simulink model "simulation"  (R2020a)
settings: Solver=VariableStepAuto  StartTime=0.0  StopTime=1200  RelTol=1e-3
values from neighbouring files (symbols this model uses):
  CHR1_Kp = 0.6/k/a    (= 0.258906601048)    [code.m]
  CHR1_Td = 0.5*Td    (= 7.8)    [code.m]
  CHR1_Ti = Td    (= 15.6)    [code.m]
  CHR2_Kp = 0.95/k/a    (= 0.40993545166)    [code.m]
  CHR2_Td = 0.42*Td    (= 6.552)    [code.m]
  CHR2_Ti = 2.38*Td    (= 37.128)    [code.m]
  k = 7.19    [code.m]
  T = 48.4    [code.m]
  Td = 15.6    [code.m]
  ZN_Kp = 1.2/k/a    (= 0.517813202097)    [code.m]
  ZN_Td = 0.5*Td    (= 7.8)    [code.m]
  ZN_Ti = 2*Td    (= 31.2)    [code.m]
undefined symbols (not defined in the file or in its folder): sigbuilder_block
settings Model: Creator=AMIRHOSEIN  LastModifiedBy=AMIRHOSEIN

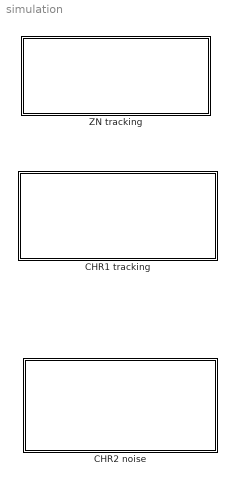
== system simulation ==
  CHR1 tracking : Subsystem
  CHR2 noise : Subsystem
  ZN tracking : Subsystem

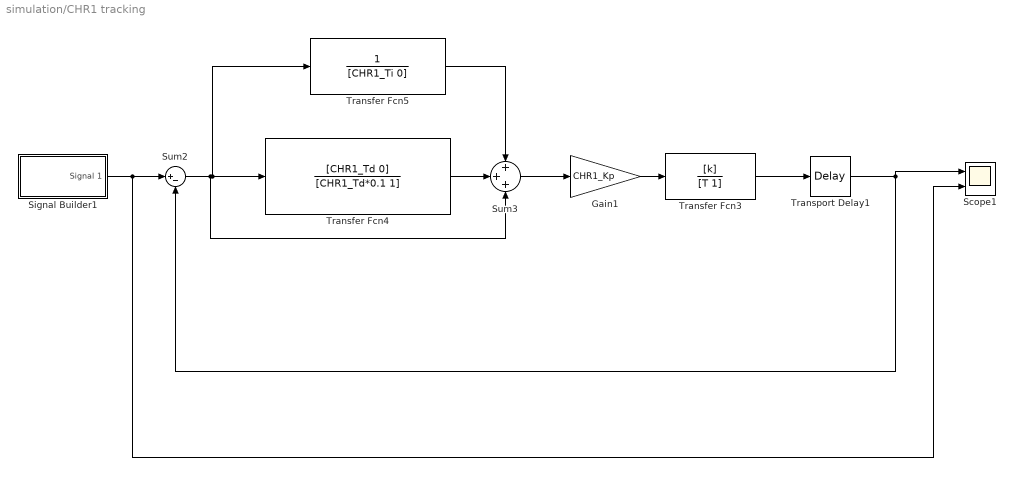
== system simulation/CHR1 tracking ==
  Gain1 : Gain  Gain=CHR1_Kp
  Scope1 : Scope  NumInputPorts=2
  Signal Builder1 : Subsystem  Tag=STV Subsys  LoadFcn=sigbuilder_block('load');  StartFcn=sigbuilder_block('start');  StopFcn=sigbuilder_block('stop');  ClipboardFcn=sigbuilder_block('clipboard');  mask(Sigbuilder block){tuvar=[0:10]}
      mask help: Simulink:masks:SigbuilderBlock_MD
      mask init:
      | if ~strcmp(get_param(bdroot(gcbh),'SimulationStatus'),'stopped') tuvar = sigbuilder_block('maskInit'); end
      settings: CopyFcn=sigbuilder_block('copy');  DeleteFcn=sigbuilder_block('delete');  ModelCloseFcn=sigbuilder_block('modelClose');  PreSaveFcn=sigbuilder_block('preSave');  PauseFcn=sigbuilder_block('pause');  ContinueFcn=sigbuilder_block('continue');  NameChangeFcn=sigbuilder_block('namechange');  OpenFcn=sigbuilder_block('open',[744.75 240 550.5 396 ]);  CloseFcn=sigbuilder_block('close');
      mask Display: plot(0, 0, 100, 100,[2, 2, 32, 32, 2], [68, 8, 8, 68, 68],[32, 2], [38, 38], [32, 19, 2],[53, 60, 44], [32, 17, 17, 2],[16, 16, 31, 31]);txt = getActiveGroup(gcbh);text(2, 100, txt,'verticalAlignment', 'top');
  Sum2 : Sum  Inputs=|+-
  Sum3 : Sum  Inputs=+++
  Transfer Fcn3 : TransferFcn  Numerator=[k]  Denominator=[T 1]
  Transfer Fcn4 : TransferFcn  Numerator=[CHR1_Td 0]  Denominator=[CHR1_Td*0.1 1]
  Transfer Fcn5 : TransferFcn  Denominator=[CHR1_Ti 0]
  Transport Delay1 : TransportDelay  DelayTime=Td
  wires:
  Transfer Fcn5/1 -> Sum3/1
  Transfer Fcn4/1 -> Sum3/2
  Transfer Fcn3/1 -> Transport Delay1/1
  Transport Delay1/1 -> Sum2/2, Scope1/1
  Sum2/1 -> Sum3/3, Transfer Fcn4/1, Transfer Fcn5/1
  Sum3/1 -> Gain1/1
  Gain1/1 -> Transfer Fcn3/1
  Signal Builder1/1(Signal 1) -> Scope1/2, Sum2/1

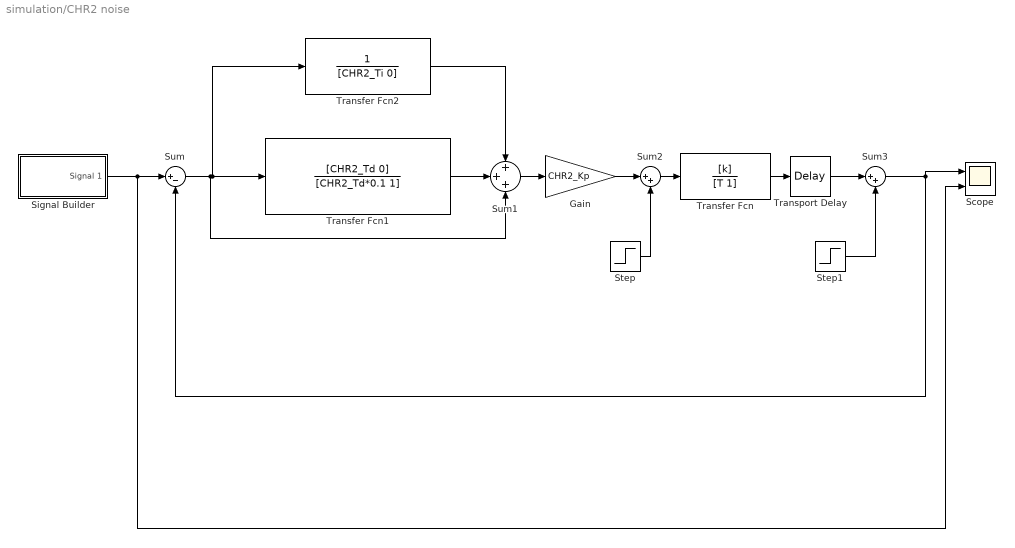
== system simulation/CHR2 noise ==
  Gain : Gain  Gain=CHR2_Kp
  Scope : Scope  NumInputPorts=2
  Signal Builder : Subsystem  Tag=STV Subsys  LoadFcn=sigbuilder_block('load');  StartFcn=sigbuilder_block('start');  StopFcn=sigbuilder_block('stop');  ClipboardFcn=sigbuilder_block('clipboard');  mask(Sigbuilder block){tuvar=[0:10]}
      mask help: Simulink:masks:SigbuilderBlock_MD
      mask init:
      | if ~strcmp(get_param(bdroot(gcbh),'SimulationStatus'),'stopped') tuvar = sigbuilder_block('maskInit'); end
      settings: CopyFcn=sigbuilder_block('copy');  DeleteFcn=sigbuilder_block('delete');  ModelCloseFcn=sigbuilder_block('modelClose');  PreSaveFcn=sigbuilder_block('preSave');  PauseFcn=sigbuilder_block('pause');  ContinueFcn=sigbuilder_block('continue');  NameChangeFcn=sigbuilder_block('namechange');  OpenFcn=sigbuilder_block('open',[538.5 220.5 550.5 396 ]);  CloseFcn=sigbuilder_block('close');
      mask Display: plot(0, 0, 100, 100,[2, 2, 32, 32, 2], [68, 8, 8, 68, 68],[32, 2], [38, 38], [32, 19, 2],[53, 60, 44], [32, 17, 17, 2],[16, 16, 31, 31]);txt = getActiveGroup(gcbh);text(2, 100, txt,'verticalAlignment', 'top');
  Step : Step  Time=600  After=10  SampleTime=0
  Step1 : Step  Time=1000  After=10  SampleTime=0
  Sum : Sum  Inputs=|+-
  Sum1 : Sum  Inputs=+++
  Sum2 : Sum  Inputs=|++
  Sum3 : Sum  Inputs=|++
  Transfer Fcn : TransferFcn  Numerator=[k]  Denominator=[T 1]
  Transfer Fcn1 : TransferFcn  Numerator=[CHR2_Td 0]  Denominator=[CHR2_Td*0.1 1]
  Transfer Fcn2 : TransferFcn  Denominator=[CHR2_Ti 0]
  Transport Delay : TransportDelay  DelayTime=Td
  wires:
  Signal Builder/1(Signal 1) -> Scope/2, Sum/1
  Step/1 -> Sum2/2
  Sum2/1 -> Transfer Fcn/1
  Sum3/1 -> Sum/2, Scope/1
  Transport Delay/1 -> Sum3/1
  Transfer Fcn/1 -> Transport Delay/1
  Gain/1 -> Sum2/1
  Step1/1 -> Sum3/2
  Sum/1 -> Sum1/3, Transfer Fcn1/1, Transfer Fcn2/1
  Transfer Fcn1/1 -> Sum1/2
  Transfer Fcn2/1 -> Sum1/1
  Sum1/1 -> Gain/1

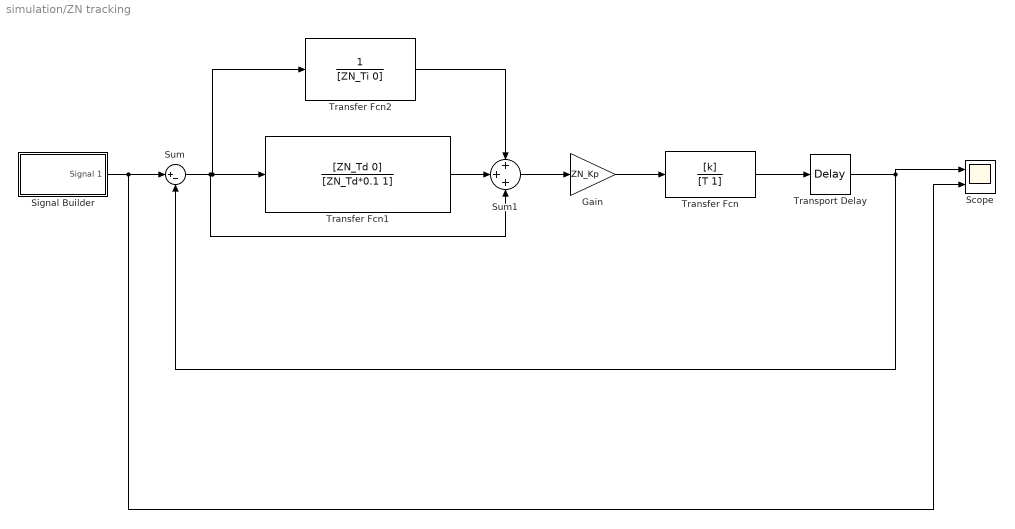
== system simulation/ZN tracking ==
  Gain : Gain  Gain=ZN_Kp
  Scope : Scope  NumInputPorts=2
  Signal Builder : Subsystem  Tag=STV Subsys  LoadFcn=sigbuilder_block('load');  StartFcn=sigbuilder_block('start');  StopFcn=sigbuilder_block('stop');  ClipboardFcn=sigbuilder_block('clipboard');  mask(Sigbuilder block){tuvar=[0:10]}
      mask help: Simulink:masks:SigbuilderBlock_MD
      mask init:
      | if ~strcmp(get_param(bdroot(gcbh),'SimulationStatus'),'stopped') tuvar = sigbuilder_block('maskInit'); end
      settings: CopyFcn=sigbuilder_block('copy');  DeleteFcn=sigbuilder_block('delete');  ModelCloseFcn=sigbuilder_block('modelClose');  PreSaveFcn=sigbuilder_block('preSave');  PauseFcn=sigbuilder_block('pause');  ContinueFcn=sigbuilder_block('continue');  NameChangeFcn=sigbuilder_block('namechange');  OpenFcn=sigbuilder_block('open',[744.75 240 550.5 396 ]);  CloseFcn=sigbuilder_block('close');
      mask Display: plot(0, 0, 100, 100,[2, 2, 32, 32, 2], [68, 8, 8, 68, 68],[32, 2], [38, 38], [32, 19, 2],[53, 60, 44], [32, 17, 17, 2],[16, 16, 31, 31]);txt = getActiveGroup(gcbh);text(2, 100, txt,'verticalAlignment', 'top');
  Sum : Sum  Inputs=|+-
  Sum1 : Sum  Inputs=+++
  Transfer Fcn : TransferFcn  Numerator=[k]  Denominator=[T 1]
  Transfer Fcn1 : TransferFcn  Numerator=[ZN_Td 0]  Denominator=[ZN_Td*0.1 1]
  Transfer Fcn2 : TransferFcn  Denominator=[ZN_Ti 0]
  Transport Delay : TransportDelay  DelayTime=Td
  wires:
  Transport Delay/1 -> Sum/2, Scope/1
  Transfer Fcn2/1 -> Sum1/1
  Sum/1 -> Sum1/3, Transfer Fcn1/1, Transfer Fcn2/1
  Transfer Fcn/1 -> Transport Delay/1
  Sum1/1 -> Gain/1
  Transfer Fcn1/1 -> Sum1/2
  Gain/1 -> Transfer Fcn/1
  Signal Builder/1(Signal 1) -> Scope/2, Sum/1

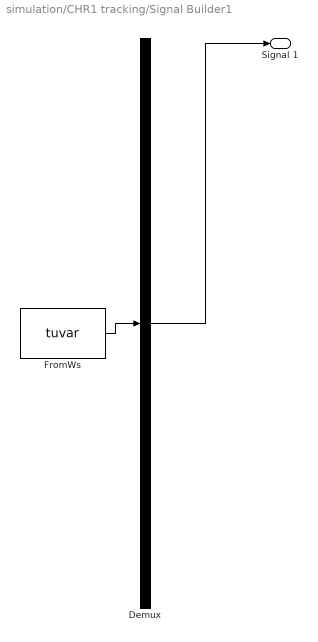
== system simulation/CHR1 tracking/Signal Builder1 ==
  Demux : Demux  Tag=STV Demux  Outputs=1
      settings: DisplayOption=none
  FromWs : FromWorkspace  Tag=STV FromWs  VariableName=tuvar
      SigBuilderData=|
      | common.afterFinalStr = 'Extrapolate'
      | common.sampleTime = 0
      | dataSet.timeRange = [0 1200]
      | dataSet.name = 'Group 1'
      | sbobj.Groups.Name = 'Group 1'
      | sbobj.Groups.Signals.Name = 'Signal 1'
      | sbobj.Groups.Signals.XData = [0 400 400 800 800 1200]
      | sbobj.Groups.Signals.YData = [35 35 55 55 45 45]
      | sbobj.Groups.TimeRange = [0 1200]
  Signal 1 : Outport  Tag=STV Outport
  wires:
  Demux/1 -> Signal 1/1
  FromWs/1 -> Demux/1

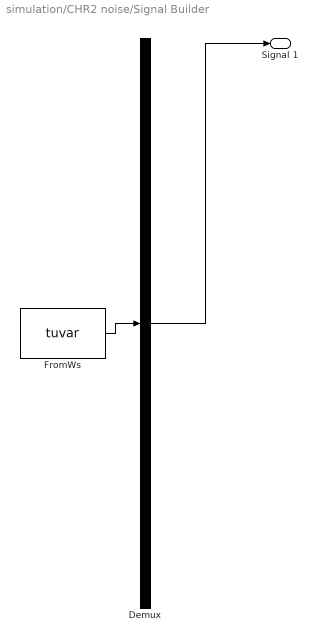
== system simulation/CHR2 noise/Signal Builder ==
  Demux : Demux  Tag=STV Demux  Outputs=1
      settings: DisplayOption=none
  FromWs : FromWorkspace  Tag=STV FromWs  VariableName=tuvar
      SigBuilderData=|
      | common.afterFinalStr = 'Extrapolate'
      | common.sampleTime = 0
      | dataSet.timeRange = [0 1200]
      | dataSet.name = 'Group 1'
      | sbobj.Groups.Name = 'Group 1'
      | sbobj.Groups.Signals.Name = 'Signal 1'
      | sbobj.Groups.Signals.XData = [0 400 400 800 800 1200]
      | sbobj.Groups.Signals.YData = [35 35 55 55 45 45]
      | sbobj.Groups.TimeRange = [0 1200]
  Signal 1 : Outport  Tag=STV Outport
  wires:
  Demux/1 -> Signal 1/1
  FromWs/1 -> Demux/1

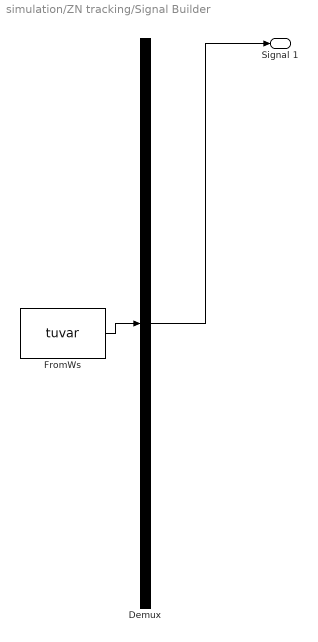
== system simulation/ZN tracking/Signal Builder ==
  Demux : Demux  Tag=STV Demux  Outputs=1
      settings: DisplayOption=none
  FromWs : FromWorkspace  Tag=STV FromWs  VariableName=tuvar
      SigBuilderData=|
      | common.afterFinalStr = 'Extrapolate'
      | common.sampleTime = 0
      | dataSet.timeRange = [0 1200]
      | dataSet.name = 'Group 1'
      | sbobj.Groups.Name = 'Group 1'
      | sbobj.Groups.Signals.Name = 'Signal 1'
      | sbobj.Groups.Signals.XData = [0 400 400 800 800 1200]
      | sbobj.Groups.Signals.YData = [35 35 55 55 45 45]
      | sbobj.Groups.TimeRange = [0 1200]
  Signal 1 : Outport  Tag=STV Outport
  wires:
  Demux/1 -> Signal 1/1
  FromWs/1 -> Demux/1
